simulink model "sf_launchabort"  (R2017b)
settings: Solver=FixedStepDiscrete  StartTime=0.0  StopTime=136  RelTol=1e-3
undefined symbols (not defined in the file): sigbuilder_block
libraries: vrlib x2
settings Model: Creator=The MathWorks, Inc.  LastModifiedBy=The MathWorks, Inc.
settings DataIOCC: LimitDataPoints=on  SaveFormat=Array
settings OptimizationCC: ExpressionDepthLimit=2147483647  InitFltsAndDblsToZero=on  EfficientMapNaN2IntZero=off  LifeSpan=1
settings DebuggingCC: SaveWithParameterizedLinksMsg=none  UnderspecifiedInitializationDetection=Classic  MergeDetectMultiDrivingBlocksExec=none  SignalResolutionControl=TryResolveAllWithWarning  FcnCallInpInsideContextMsg=warning  StateNameClashWarn=warning  StrictBusMsg=Warning  SFUnexpectedBacktrackingDiag=warning  SFNoUnconditionalDefaultTransitionDiag=warning  SFExecutionAtInitializationDiag=none
settings HardwareCC: ProdBitPerPointer=32  ProdBitPerSizeT=32  ProdBitPerPtrDiffT=32  ProdLargestAtomicFloat=None  ProdIntDivRoundTo=Undefined  ProdEndianess=Unspecified  ProdWordSize=32  ProdHWDeviceType=32-bit Generic
settings ModelReferenceCC: PropagateSignalLabelsOutOfModel=off
settings SFSimCC: SimParseCustomCode=off
settings RTWCC: SystemTargetFile=ert.tlc  GenCodeOnly=on  TemplateMakefile=ert_default_tmf  Description=Real-Time Workshop Embedded Coder (no auto configuration)  GenerateReport=on  IncludeHyperlinkInReport=on  LaunchReport=on
settings CodeAppCC: IgnoreCustomStorageClasses=off  CustomSymbolStrGlobalVar=$N$M  CustomSymbolStrType=$N$M  CustomSymbolStrFcn=$N$M$F  CustomSymbolStrModelFcn=$N  CustomSymbolStrMacro=$N$M  StateflowObjectComments=on  InternalIdentifier=Classic
settings ERTTargetCC: TargetFcnLib=ansi_tfl_tmw.mat  MultiwordLength=2048  GenerateSampleERTMain=on  SupportContinuousTime=on  ERTCustomFileTemplate=example_file_process.tlc  ConvertIfToSwitch=off  SuppressUnreachableDefaultCases=off
settings ConfigComp: CovScope=Subsystem  CovPath=/launchAbortController  CovMetricSettings=dcmrw  CovHtmlReporting=on  CovSaveCumulativeToWorkspaceVar=on  CovSaveSingleToWorkspaceVar=on  CovExternalEMLEnable=off

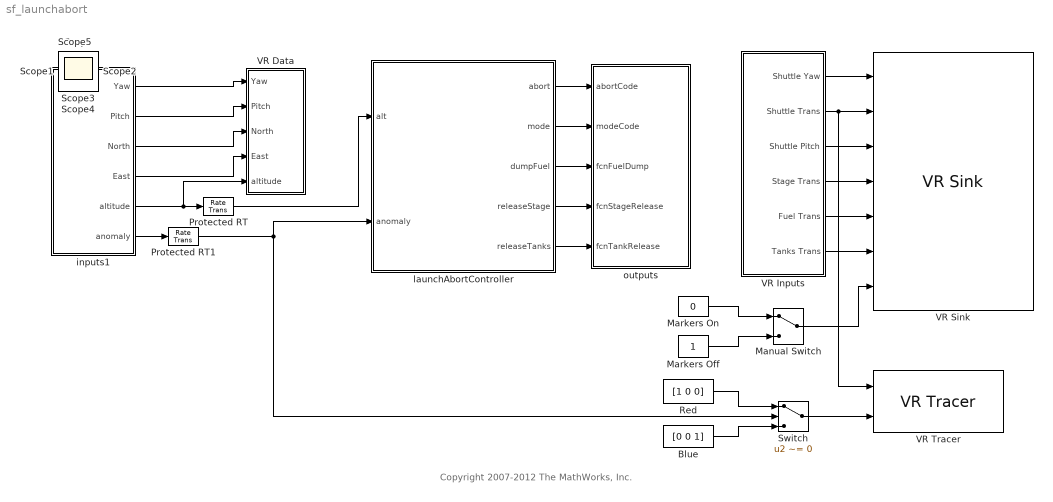
== system sf_launchabort ==
  note: Copyright 2007-2012 The MathWorks, Inc.
  Blue : Constant  Value=[0 0 1]
  Manual Switch : ManualSwitch
  Markers Off : Constant
  Markers On : Constant  Value=0
  Protected RT : RateTransition  Deterministic=off
  Protected RT1 : RateTransition  Deterministic=off
  Red : Constant  Value=[1 0 0]
  Switch : Switch  Criteria=u2 ~= 0
  VR Data : Subsystem
  VR Inputs : Subsystem
  VR Sink : vrlib/VR Sink  InstantiateOnLoad=on  SampleTime=0.1  ViewEnable=on  RemoteChange=off  RemoteView=on  FieldsWritten=ShuttleYaw.rotation.4.1.double#ShuttleYaw.translation.3.1.double#ShuttlePitch.rotation.4.1.double#StageYaw.translation.3.1.double#dumpedFuel.translation.3.1.double#TanksYaw.translation.3.1.double#Marker_Switch.whichChoice.1.1.double  WorldFileName=abortVR.wrl  WorldDescription=Launch Abort - VR  AutoView=on  VideoDimensions=[]  AllowVariableSize=off  FigureProperties="{'Position', 'Name', 'Viewpoint', 'CameraBound', 'CameraDirection', 'CameraPosition', 'CameraUpVector', 'ZoomFactor', 'Antialiasing', 'Headlight', 'Lighting', 'NavPanel', 'Sound', 'StatusBar', 'Stereo3D', 'Stereo3DCameraOffset', 'Stereo3DHIT', 'ToolBar', 'Textures', 'Transparency', 'Triad', 'Wireframe', 'NavZones', 'NavMode', 'NavSpeed', 'CaptureFileFormat', 'CaptureFileName', 'Record2DCompressMethod', 'Record2DCompressQuality', 'Record2D', 'Record2DFileName', 'Record2DFPS'; [1.1100000000000000e+02   2.6400000000000000e+02   5.8600000000000000e+02   4.0600000000000000e+02], 'Launch Abort - VR', 'Chase Plane', 'on', [0.0000000000000000e+00   0.0000000000000000e+00  -1.0000000000000000e+00], [0.0000000000000000e+00   0.0000000000000000e+00   0.0000000000000000e+00], [0.0000000000000000e+00   1.0000000000000000e+00   0.0000000000000000e+00], [1.0000000000000000e+00], 'on', 'on', 'on', 'halfbar', 'on', 'on', 'off', [1.0000000149011612e-01], [0.0000000000000000e+00], 'on', 'on', 'on', 'none', 'off', 'off', 'examine', 'veryslow', 'tif', '%f_anim_%n.tif', 'auto', [7.5000000000000000e+01], 'off', '%f_anim_%n.avi', [1.5000000000000000e+01]}"
      settings: SourceProductBaseCode=VR
  VR Tracer : vrlib/VR Tracer  VrmlFile=abortVR.wrl  ParentNode=Markers  MarkerName=Tetrahedron  UseLines=off  UseTriads=off  MarkerScale=[20 20 20]  MarkerColorSelection=Block input  MarkerColor=red  rgbval=[1 0 0]  Ts=1  ForceViewerOpen=off  ConnectPlane=off  PlaneCoeff=[0 1 0 0]  ConnectPoint=None  PointCoord=[0 0 0]
      settings: SourceProductName=Simulink 3D Animation  SourceProductBaseCode=VR
  inputs1 : Subsystem  Tag=STV Subsys  LoadFcn=sigbuilder_block('load');  StartFcn=sigbuilder_block('start');  StopFcn=sigbuilder_block('stop');  ClipboardFcn=sigbuilder_block('clipboard');  mask(Sigbuilder block){tuvar=[0:10]}
      mask help: Sigbuilder GUI
      mask init:
      | if ~strcmp(get_param(bdroot(gcbh),'SimulationStatus'),'stopped') tuvar = sigbuilder_block('maskInit'); end
      settings: CopyFcn=sigbuilder_block('copy');  DeleteFcn=sigbuilder_block('delete');  ModelCloseFcn=sigbuilder_block('modelClose');  PreSaveFcn=sigbuilder_block('preSave');  PauseFcn=sigbuilder_block('pause')  ContinueFcn=sigbuilder_block('continue')  NameChangeFcn=sigbuilder_block('namechange');  OpenFcn=sigbuilder_block('open',[81 93.75 561 399.75 ]);  CloseFcn=sigbuilder_block('close');
      mask Display: plot(0, 0, 100, 100,[2, 2, 32, 32, 2], [68, 8, 8, 68, 68],[32, 2], [38, 38], [32, 19, 2],[53, 60, 44], [32, 17, 17, 2],[16, 16, 31, 31]);txt = getActiveGroup(gcbh);text(2, 100, txt,'verticalAlignment', 'top');
  launchAbortController : Stateflow chart  TreatAsAtomicUnit=on
      settings: RTWSystemCode=Reusable function  RTWFcnNameOpts=Use subsystem name  RTWFileNameOpts=Use subsystem name
  outputs : Subsystem
  Scope{,1..5} (6 alike) : Scope
  wires:
  launchAbortController/1(abort) -> outputs/1(abortCode)
  launchAbortController/2(mode) -> outputs/2(modeCode)
  launchAbortController/3(dumpFuel) -> outputs/3(fcnFuelDump)
  launchAbortController/4(releaseStage) -> outputs/4(fcnStageRelease)
  launchAbortController/5(releaseTanks) -> outputs/5(fcnTankRelease)
  VR Inputs/2(Shuttle Trans) -> VR Sink/2, VR Tracer/1
  inputs1/5(altitude) -> Protected RT/1, VR Data/5(altitude)
  inputs1/4(East) -> VR Data/4(East)
  inputs1/3(North) -> VR Data/3(North)
  inputs1/2(Pitch) -> VR Data/2(Pitch)
  inputs1/1(Yaw) -> VR Data/1(Yaw)
  inputs1/6(anomaly) -> Protected RT1/1
  Protected RT/1 -> launchAbortController/1(alt)
  Protected RT1/1 -> launchAbortController/2(anomaly), Switch/2
  Red/1 -> Switch/1
  Blue/1 -> Switch/3
  VR Inputs/1(Shuttle Yaw) -> VR Sink/1
  VR Inputs/3(Shuttle Pitch) -> VR Sink/3
  VR Inputs/4(Stage Trans) -> VR Sink/4
  VR Inputs/5(Fuel Trans) -> VR Sink/5
  VR Inputs/6(Tanks Trans) -> VR Sink/6
  Markers On/1 -> Manual Switch/1
  Markers Off/1 -> Manual Switch/2
  Manual Switch/1 -> VR Sink/7
  Switch/1 -> VR Tracer/2

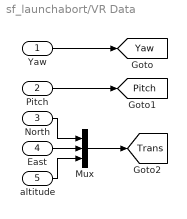
== system sf_launchabort/VR Data ==
  Yaw : Inport
  Pitch : Inport  Port=2
  North : Inport  Port=3
  East : Inport  Port=4
  altitude : Inport  Port=5
  Mux : Mux  Inputs=3
  tag scope: Pitch=global, Trans=global, Yaw=global
  wires:
  East/1 -> Mux/2
  North/1 -> Mux/1
  Pitch/1 -> [Pitch]
  Yaw/1 -> [Yaw]
  altitude/1 -> Mux/3
  Mux/1 -> [Trans]

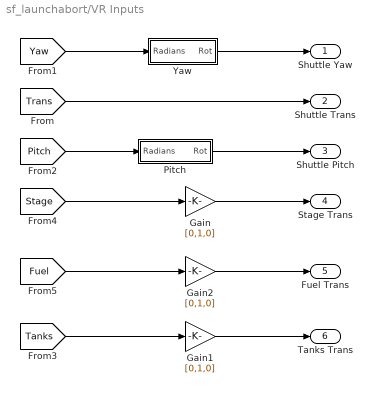
== system sf_launchabort/VR Inputs ==
  Gain : Gain  Gain=[0,1,0]
  Gain1 : Gain  Gain=[0,1,0]
  Gain2 : Gain  Gain=[0,1,0]
  Pitch : Subsystem  mask{axisRot=X}
      mask prompts: axisRot "Axis of Rotation"
      mask TypeOptions axisRot: X | Y | Z
      mask Callback axisRot:
      | constantBlock = [gcb, '/rotVector'];
      | switch get_param(gcb, 'axisRot'),
      |     case('X'),
      |         set_param(constantBlock, 'Value', '[1, 0, 0]');
      |     case('Y'),
      |         set_param(constantBlock, 'Value', '[0, 1, 0]');
      |     case('Z'),
      |         set_param(constantBlock, 'Value', '[0, 0, 1]');
      | end
      | clear constantBlock;
  Yaw : Subsystem  mask{axisRot=Z}
      mask prompts: axisRot "Axis of Rotation"
      mask TypeOptions axisRot: X | Y | Z
      mask Callback axisRot:
      | constantBlock = [gcb, '/rotVector'];
      | switch get_param(gcb, 'axisRot'),
      |     case('X'),
      |         set_param(constantBlock, 'Value', '[1, 0, 0]');
      |     case('Y'),
      |         set_param(constantBlock, 'Value', '[0, 1, 0]');
      |     case('Z'),
      |         set_param(constantBlock, 'Value', '[0, 0, 1]');
      | end
      | clear constantBlock;
  Shuttle Yaw : Outport
  Shuttle Trans : Outport  Port=2
  Shuttle Pitch : Outport  Port=3
  Stage Trans : Outport  Port=4
  Fuel Trans : Outport  Port=5
  Tanks Trans : Outport  Port=6
  wires:
  [Trans] -> Shuttle Trans/1
  [Tanks] -> Gain1/1
  [Yaw] -> Yaw/1(Radians)
  [Pitch] -> Pitch/1(Radians)
  Pitch/1(Rot) -> Shuttle Pitch/1
  Yaw/1(Rot) -> Shuttle Yaw/1
  Gain/1 -> Stage Trans/1
  Gain1/1 -> Tanks Trans/1
  [Stage] -> Gain/1
  [Fuel] -> Gain2/1
  Gain2/1 -> Fuel Trans/1

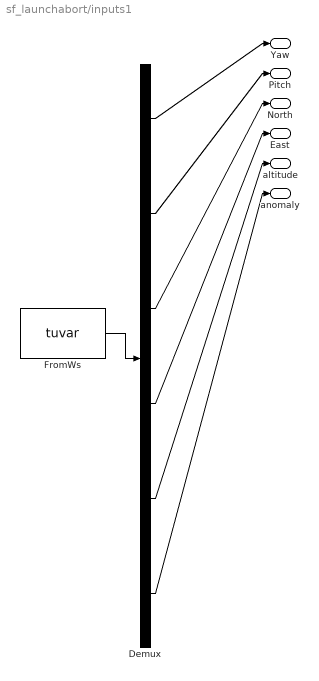
== system sf_launchabort/inputs1 ==
  Demux : Demux  Tag=STV Demux  Outputs=6
  FromWs : FromWorkspace  Tag=STV FromWs  VariableName=tuvar  SampleTime=0
  Yaw : Outport  Tag=STV Outport
  Pitch : Outport  Tag=STV Outport  Port=2
  North : Outport  Tag=STV Outport  Port=3
  East : Outport  Tag=STV Outport  Port=4
  altitude : Outport  Tag=STV Outport  Port=5
  anomaly : Outport  Tag=STV Outport  Port=6
  wires:
  Demux/6 -> anomaly/1
  Demux/5 -> altitude/1
  Demux/4 -> East/1
  Demux/3 -> North/1
  Demux/2 -> Pitch/1
  Demux/1 -> Yaw/1
  FromWs/1 -> Demux/1

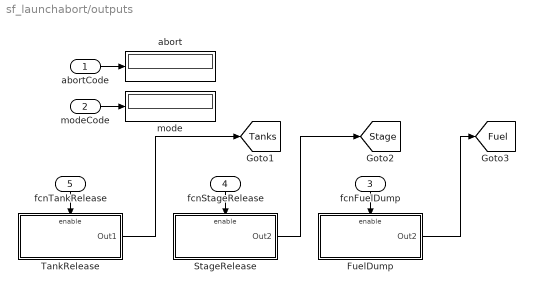
== system sf_launchabort/outputs ==
  abortCode : Inport
  modeCode : Inport  Port=2
  fcnFuelDump : Inport  Port=3
  fcnStageRelease : Inport  Port=4
  fcnTankRelease : Inport  Port=5
  FuelDump : Subsystem  TreatAsAtomicUnit=on
  StageRelease : Subsystem  TreatAsAtomicUnit=on
  TankRelease : Subsystem  TreatAsAtomicUnit=on
  abort : Display
  mode : Display
  tag scope: Fuel=global, Stage=global, Tanks=global
  wires:
  abortCode/1 -> abort/1
  modeCode/1 -> mode/1
  fcnFuelDump/1 -> FuelDump/Enable
  fcnStageRelease/1 -> StageRelease/Enable
  fcnTankRelease/1 -> TankRelease/Enable
  StageRelease/1(Out2) -> [Stage]
  TankRelease/1(Out1) -> [Tanks]
  FuelDump/1(Out2) -> [Fuel]

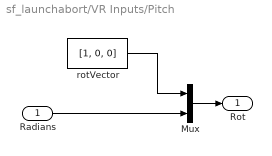
== system sf_launchabort/VR Inputs/Pitch ==
  Radians : Inport
  Mux : Mux  Inputs=2
  rotVector : Constant  Value=[1, 0, 0]
  Rot : Outport
  wires:
  Radians/1 -> Mux/2
  rotVector/1 -> Mux/1
  Mux/1 -> Rot/1

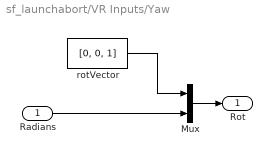
== system sf_launchabort/VR Inputs/Yaw ==
  Radians : Inport
  Mux : Mux  Inputs=2
  rotVector : Constant  Value=[0, 0, 1]
  Rot : Outport
  wires:
  Radians/1 -> Mux/2
  rotVector/1 -> Mux/1
  Mux/1 -> Rot/1

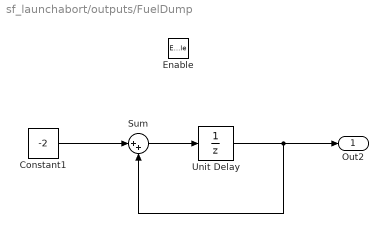
== system sf_launchabort/outputs/FuelDump ==
  Enable : EnablePort
  Constant1 : Constant  Value=-2
  Sum : Sum  Inputs=|++
  Unit Delay : UnitDelay  SampleTime=-1
  Out2 : Outport  InitialOutput=0
  wires:
  Unit Delay/1 -> Sum/2, Out2/1
  Sum/1 -> Unit Delay/1
  Constant1/1 -> Sum/1

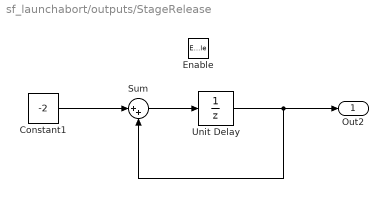
== system sf_launchabort/outputs/StageRelease ==
  Enable : EnablePort
  Constant1 : Constant  Value=-2
  Sum : Sum  Inputs=|++
  Unit Delay : UnitDelay  SampleTime=-1
  Out2 : Outport  InitialOutput=0
  wires:
  Unit Delay/1 -> Sum/2, Out2/1
  Sum/1 -> Unit Delay/1
  Constant1/1 -> Sum/1

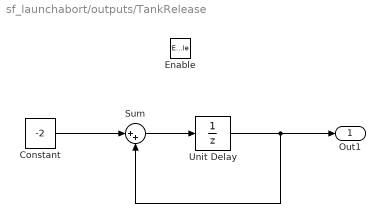
== system sf_launchabort/outputs/TankRelease ==
  Enable : EnablePort
  Constant : Constant  Value=-2
  Sum : Sum  Inputs=|++
  Unit Delay : UnitDelay  SampleTime=-1
  Out1 : Outport  InitialOutput=0
  wires:
  Unit Delay/1 -> Out1/1, Sum/2
  Constant/1 -> Sum/1
  Sum/1 -> Unit Delay/1

== stateflow chart sf_launchabort/launchAbortController ==
  settings: updateMethod=DISCRETE  sampleTime=1
  state ModeLogic [parallel]
    settings: executionOrder=1
    state RTLS
      entry:mode=1;
    state DRL
      entry:mode=2;
    state ATO
      entry:mode=4;
    state AOA
      entry:mode=3;
    (default) -> RTLS
    RTLS -> DRL : [alt>10000 && !anomaly]
    DRL -> AOA : [alt>100000 && !anomaly]
    AOA -> ATO : [alt>400000 && !anomaly]
  state Abort [parallel]
    settings: executionOrder=2
    state Normal
      en: abort=NO_ABORT;
    state abortLogic
      en: abort = ABORT_STARTED;
      state FuelDump
        dumpFuel;
        ex: abort=FUEL_DUMP_DONE;
      state TankRelease
        releaseTanks;
        ex: abort=TANK_RELEASE_DONE;
      state StageRelease
        releaseStage;
        ex: abort=STAGE_RELEASE_DONE;
      (junction 31) -> FuelDump [order 1] : [in(ModeLogic.RTLS)]
      FuelDump -> TankRelease : after(10, tick)
      (junction 31) -> TankRelease [order 2] : [in(ModeLogic.DRL)]
      (junction 31) -> StageRelease [order 3] : [in(ModeLogic.AOA)]
      (junction 31) -> (junction 32) [order 4]
      TankRelease -> StageRelease : after(10, tick)
      StageRelease -> (junction 32)
    state abortComplete
      en: abort=ABORT_COMPLETE;
    (default) -> Normal
    Normal -> (junction 31) : [anomaly]
    (junction 32) -> abortComplete
  data: alt input; anomaly input; abort output double; mode output double; ABORT_COMPLETE constant double =5; ABORT_STARTED constant double =1; FUEL_DUMP_DONE constant double =2; NO_ABORT constant double =0; STAGE_RELEASE_DONE constant double =4; TANK_RELEASE_DONE constant double =3
  events: dumpFuel output EITHER_EDGE_EVENT; releaseStage output EITHER_EDGE_EVENT; releaseTanks output EITHER_EDGE_EVENT
